simulink model "dspvorbisdec"  (Simulink 8.3)
settings: Solver=FixedStepDiscrete  SolverMode=SingleTasking  StartTime=0.0  StopTime=inf  RelTol=1e-3
PostLoadFcn:
  | hws  = get_param(bdroot,'modelworkspace');
  | dspvorbisdec_SampRt = hws.evalin('dspvorbisdec_OutputSampRt');
  | clear hws;
StopFcn:
  | dspvorbisdec_hws = get_param(bdroot,'modelworkspace');
  | dspvorbisdec_tmp = dspvorbisdec_hws.data;
  | for i = 1:length(dspvorbisdec_tmp)
  |   if strcmp(dspvorbisdec_tmp(i).Name,'dspvorbisdec_OutputSampRt')
  |      if (dspvorbisdec_tmp(i).Value~=dspvorbisdec_SampRt)
  |         dspvorbisdec_hws.assignin('dspvorbisdec_OutputSampRt', dspvorbisdec_SampRt);
  |      end
  |   end
  | end
  | 
  | clear hws dspvorbisdec_tmp i dspvorbisdec_hws;
undefined symbols (not defined in the file or in its folder): blockSize, errordlg, uiwait, warndlg
libraries: simulink x5, dspmtrx3 x3, dspindex x2, dspsigops x1, dspxfrm3 x1, dspmisc x1, dspsnks4 x1, dspsrcs4 x1
(part 3 of 3)

== matlab function Decode All Pages of Data/decodePage/Read Setup Info/Read Setup ==
  data: data input double; codeBooks output double; floor1Data output double; floor1DataLocs output double; resiData output double; numBytes input double; ifUnpack input double; resiDataLocs output double; mapData output double; modeData output double; numChannels input double
function [codeBooks, floor1Data, floor1DataLocs, resiData, resiDataLocs, mapData, modeData] = readSetup(data, numBytes, ifUnpack, numChannels)

codeBooks = uint32(zeros(2*64, 256*30)); % reserve space for codebooks. Standard has capacity for up to 2^32 of them. 
                                         % In this model we assume that number of codebooks cannot be more than 64. Change this quanitity if out of bounds error is experienced
dimLocs = uint32(zeros(256,1));           % Auxiliary array. To specify location of different data in a storage vector
floor1Data = uint32(zeros(256,1));
floor1DataLocs = uint32(zeros(5,32));   % Auxiliary array for floor data vector
resiData = uint32(zeros(256*2,1)); 
resiDataLocs = uint32(zeros(2,8));    % Auxiliary array for residue data vector
mapData = uint32(zeros(5,8));           % Assume we have no more than 2-channel audio
modeData = uint32(zeros(32,1));           % (Same)

persistent tmpPoint;
if isempty(tmpPoint)
	tmpPoint = uint16(0);
end
persistent tmpStorage;
if isempty(tmpStorage)
    tmpStorage = uint32(zeros(15000,1));
end


% Here we check whether compressed setup info header has been buffered completely (ifUnpack==1), 
% or otherwise (ifUnpack==0). 
if (~ifUnpack)
    % If the buffering is not complete yet, then write the first page into temporary buffer
    for w = 1:numBytes
        tmpStorage(tmpPoint+w) = data(w);
    end
    tmpPoint = tmpPoint+numBytes;
else
    % Concatenate the previous page of compressed setup header with the current one and proceed to decoding
    bitstr = logical(false(120000,1));
    for m = 1:tmpPoint
        for t = eml.unroll(1:8)
            bitstr(8*(m-1)+t) = bitget(tmpStorage(m), t);
        end
    end
    for m = 1:numBytes
        for t = eml.unroll(1:8)
            bitstr(8*(m-1)+t+tmpPoint*8) = bitget(data(m), t);
        end
    end
    tmpPoint = uint16(0);    

    %%%%%%%%%%%%%%%%%%%%%%%%%%%%%%%%%%%%%%%%%%%%%%%%%
    %% The code below follows Vorbis decoder spec. %%
    %%%%%%%%%%%%%%%%%%%%%%%%%%%%%%%%%%%%%%%%%%%%%%%%%

    sHead = zeros(3,8);
    tmp = uint8([66 67 86]'); %%%%% Codebook starts with a sync pattern
    for i = uint32(1):uint32(3)
        sHead(i,:) = bitget(tmp(i),1:8);
    end
    syncHead = uint32(reshape(sHead', 24,1));

    %%%%%% Skipping 'Packet type' and 'v o r b i s' fields, 7 bytes total
    bitPoint = uint32(8)*uint32(7) + uint32(1);

    countBooks = uint32(1);
    bitPoint = bitPoint+8;

    % Loop until all codebooks are read 
    totalBooks = uint32(255); %%%%% To be updated
    while (countBooks<=totalBooks)
        codeBook = uint32(zeros(256*30, 1));
    %%%%% We are looking for the sync pattern first
        a = bitPoint;
        while (1==1)
            res=uint32(1);
            i1 = uint32(1):uint32(24);
            i2 = i1+a-1;
            if any(int8(bitstr(i2))-int8(syncHead(i1)))
                res = uint32(0);
            end
            if res; break; end;
            a = a+1;
        end
        if (countBooks ==1)
            bitPoint = a-8; %%%% Skip Sync pattern
            totalBooks = uint32(0);
            for ix = bitPoint:bitPoint+7
                totalBooks = bitset(totalBooks, ix-bitPoint+1, bitstr(ix));
            end
            totalBooks = totalBooks+1;
        end
        bitPoint = a+24;    

        %%% Read codebook dimensions
        for ix = bitPoint:bitPoint+15
            codeBook(1) = bitset(codeBook(1), ix-bitPoint+1, bitstr(ix));            
        end
        bitPoint = bitPoint+16;
        %%% Read codebook length
        %%% Note: can be very long 2^16 bytes. We don't consider such cases here. Assume codebook is short, a couple of kbytes.
        for ix = bitPoint:bitPoint+23
            codeBook(2) = bitset(codeBook(2), ix-bitPoint+1, bitstr(ix));                        
        end
        bitPoint = bitPoint+24;
        bytePoint = uint32(3);

        %%% Read 'ORDERED' flag
        bitPoint=bitPoint+1;
        if bitstr(bitPoint-1)
            curLength = uint32(0);
            for ix = bitPoint:bitPoint+4
                curLength = bitset(curLength, ix-bitPoint+1, bitstr(ix));                            
            end
            bitPoint = bitPoint+5;
            curLength = curLength+1;
            curEntry = uint32(0);
            while(curEntry<codeBook(2))
                ret = uint32(0);
                v = codeBook(2) - curEntry;
                while (v)
                    ret = ret+1;
                    v = bitshift(v,-1);
                end
                %%%%%%%%%%%%%%%%%%        
                number = uint32(0);
                for ix = bitPoint:bitPoint+ret-1;
                    number = bitset(number, ix-bitPoint+1, bitstr(ix));                                                
                end
                bitPoint = bitPoint+ret; % Write entries, ordered
                for k = curEntry:(curEntry+number-1)
                    codeBook(bytePoint) = curLength;
                    bytePoint = bytePoint + 1;
                end
                curEntry = curEntry + number;
                curLength = curLength + 1;
            end
        else
            %%% Read 'SPARSE' flag
            bitPoint=bitPoint+1;       
            if bitstr(bitPoint-1) %% Read entries, sparse
                for i = uint32(1):codeBook(2)
                    bitPoint = bitPoint+1;                
                    if bitstr(bitPoint-1)
                        for ix = bitPoint:bitPoint+4
                            codeBook(bytePoint) = bitset(codeBook(bytePoint), ix-bitPoint+1, bitstr(ix));                                                
                        end
                        bitPoint = bitPoint + 5;
                        codeBook(bytePoint) = codeBook(bytePoint)+1;
                        bytePoint = bytePoint+1;
                    else
                        codeBook(bytePoint) = uint32(0);
                        bytePoint = bytePoint+1;
                    end
                end
            else %% Read entries, not sparse
                for i = uint32(1):codeBook(2)
                    for ix = bitPoint:bitPoint+4
                        codeBook(bytePoint) = bitset(codeBook(bytePoint), ix-bitPoint+1, bitstr(ix));                                                
                    end
                    codeBook(bytePoint) = codeBook(bytePoint)+1;                
                    bitPoint = bitPoint+5;
                    bytePoint = bytePoint+1;
                end
            end
        end

    %%%%%%%%%%%% Read VQ Lookup Header    
        for ix = bitPoint:bitPoint+3;
            codeBook(bytePoint) = bitset(codeBook(bytePoint), ix-bitPoint+1, bitstr(ix));                                                            
        end
        bitPoint = bitPoint + 4;
        bytePoint = bytePoint + 1;
        if codeBook(bytePoint-1)==0
            % Codebook is read, proceed to analysis
        else
            %%%%%%%%% Read VQ Data. Please refer to the decoder spec in 3.2.1.2 for further detail.
            for k = uint32(1):uint32(2)
                for ix = bitPoint:bitPoint+31
                    codeBook(bytePoint) = bitset(codeBook(bytePoint), ix-bitPoint+1, bitstr(ix));                                                                    
                end
                bitPoint = bitPoint + 32;
                bytePoint = bytePoint + 1;
            end            
            for ix = bitPoint:bitPoint+4
                codeBook(bytePoint) = bitset(codeBook(bytePoint), ix-bitPoint+1, bitstr(ix));                                                                
            end            
            bitPoint = bitPoint + 5;

            codeBook(bytePoint+1) = bitshift(codeBook(bytePoint),-4);            
            vqSize = uint32(bitand(codeBook(bytePoint),uint32(15)))+1;
            codeBook(bytePoint) = uint32(vqSize);
            bytePoint = bytePoint + 3;            

            if codeBook(bytePoint-6) == 1
            % The following routines were ported from the original C-code
                vals = uint32(floor(double(codeBook(2))^(1.0/double(codeBook(1))))); %%%%%%% SHOULD BE CHANGED FOR FIXPOINT IMPLEMENTATION
                while (1 == 1)
                    acc = uint32(1);
                    acc1 = uint32(1);
                    for k = uint32(1):codeBook(1)
                        acc = acc*vals;
                        acc1 = acc1*(vals+1);
                    end
                    if (acc<=codeBook(2)) && (acc1>codeBook(2))
                        countBytes = vals; codeBook(bytePoint-1) = vals; break;
                    else
                        if (acc>codeBook(2)); vals = vals - 1;
                        else vals = vals + 1; end
                    end
                end
                 %%%%%%%%%%%%%%%%%%%%%%%%%%%%%%%%%%%%%
            else
                countBytes = codeBook(1)*codeBook(2);
                codeBook(bytePoint-1) = countBytes;
            end 
            for i =uint32(1):countBytes
                for ix = bitPoint:bitPoint+vqSize-1
                    codeBook(bytePoint) = bitset(codeBook(bytePoint), ix-bitPoint+1, bitstr(ix));                                                                    
                end
                bitPoint = bitPoint + vqSize;
                bytePoint = bytePoint + 1;                
            end
        end
    %%%%%%%%%%%% Read place holders
        if (countBooks == totalBooks)
            for ix = bitPoint:bitPoint+5
                codeBook(bytePoint) = bitset(codeBook(bytePoint), ix-bitPoint+1, bitstr(ix));                                                                
            end
            bitPoint = bitPoint + 6;
            codeBook(bytePoint) = codeBook(bytePoint) + 1;
            bitPoint = bitPoint+uint32(16)*codeBook(bytePoint);
        end

    %%%%%%%%%%%%%% Build a codebook tree. Looked up in the original Vorbis C-library %%%%%%%%%%%%%%%
        nozeros = uint32(333333*ones(256*3,1)); % Auxiliary arrays
        cb = uint32(zeros(256*3,1));
        cb2 = uint32(zeros(256*3,1));

        codeBooks(2*countBooks-1, :) = codeBook(:)';

        sparsecount = 0;
        tmp1 = uint32(0);
        for ii = uint32(1):codeBooks(2*countBooks-1,2)
            if (codeBooks(2*countBooks-1, 2+ii)==0)
                sparsecount = sparsecount + 1;
            else
                tmp1 = tmp1+1;
                codeBooks(2*countBooks, codeBooks(2*countBooks-1, 2)+tmp1) = ii;
                nozeros(tmp1) = codeBooks(2*countBooks-1, 2+ii);
                cb2(tmp1) = ii;
            end
        end

        marker = uint32(zeros(33,1));                
        count = uint32(0);
        for ii = uint32(1):codeBooks(2*countBooks-1, 2)
            length1 = codeBooks(2*countBooks-1, 2+ii);
            if (length1>0) 
                entry = marker(length1);
                count = count + 1;
                codeBooks(2*countBooks, count) = entry;
                for j1 = int32(length1):-1:int32(1)
                    if bitand(marker(j1),1)
                        if (j1==1)
                            marker(1) = marker(1) +1;
                        else
                            marker(j1) = uint32(bitshift(marker(j1-1), 1));
                        end
                        break;
                    end
                    marker(j1) = marker(j1) + 1;
                end
                for j = uint32(length1+1):uint32(32) %prune the tree
                    if (bitshift(marker(j), -1)==entry)
                        entry = marker(j);
                        marker(j) = uint32(bitshift(marker(j-1), 1));
                    else
                        break;
                    end
                end
            else
                if(sparsecount==0); count = count + 1; end
            end
        end

        % bitreverse the words
        count = uint32(1);
        for ii=uint32(1):codeBooks(2*countBooks-1, 2)
            temp = uint32(0);
            for j1 = int32(0):int32(codeBooks(2*countBooks-1, 2+ii)-1)
                temp = uint32(bitshift(temp, 1));
                temp = bitor(temp, uint32(bitand(uint32(bitshift(codeBooks(2*countBooks, count), -j1)), 1)));
            end
            if (sparsecount)
                if (codeBooks(2*countBooks-1, 2+ii))
                    codeBooks(2*countBooks, count) = temp;
                    cb(count) = temp;
                    count = count + 1;
                end
            else
                codeBooks(2*countBooks, count) = temp;
                cb(count) = temp;
                count = count + 1;
            end
        end

        % Sort the codewords according to their lengths shortest 
        % come first in order to expedite decoding lookup process
        % Also create index to avoid zero-lengths codewords
        [nozeros1, idx] = sort(nozeros);
        maxLen = uint32(0);
        codeBooks(2*countBooks-1, 256*30-32) = uint32(1);
        for ii = uint32(1):tmp1
            codeBooks(2*countBooks-1, 2+ii) = nozeros1(ii);
            codeBooks(2*countBooks, ii) = cb(idx(ii));
            codeBooks(2*countBooks, codeBooks(2*countBooks-1, 2)+ii) = cb2(idx(ii));    
            if (maxLen<nozeros1(ii))
                if (maxLen>0); codeBooks(2*countBooks-1, 256*30-32+maxLen) = ii; end
                maxLen = nozeros1(ii);
            end
        end
        codeBooks(2*countBooks-1, 256*30-32+maxLen) = tmp1+1;
        for ii = uint32(1):uint32(32)
            if codeBooks(2*countBooks-1, 256*30-32+ii)==0
                codeBooks(2*countBooks-1, 256*30-32+ii)=codeBooks(2*countBooks-1, 256*30-32+ii-1);
            end
        end

        countBooks = countBooks+1; % Codebook has been read, go to the next one    
    end


    %%%%%%%%%%%%%%%%%%%%%%%%%%%%%%%%%%%%%%%%%%%%%%%%%%%%%%%%%%%%%%%%%%%%%%%%%%%%%%%%%%%%%%%%%%%%%%%%%%%%%%
    %%%%%%%%%%%%%%%%%%%%%%%%%%%%%%%% FLOOR SETUP %%%%%%%%%%%%%%%%%%%%%%%%%%%%%%%%%%%%%%%%%%%%%%%%%%%%%%%%%
    %%%%%%%%%%%%%%%%%%%%%%%%%%%%%%%%%%%%%%%%%%%%%%%%%%%%%%%%%%%%%%%%%%%%%%%%%%%%%%%%%%%%%%%%%%%%%%%%%%%%%%

    %%% Following the routines described in  7.2.2. of the spec. Type 1 of the floor is considered.
    bytePoint = uint32(1);

    for ix = bitPoint:bitPoint+5
        floor1Data(bytePoint) = bitset(floor1Data(bytePoint), ix-bitPoint+1, bitstr(ix));                                                        
    end
    floor1Data(bytePoint) = floor1Data(bytePoint)+1;
    bitPoint = bitPoint + 6;
    totalFloor1 = floor1Data(bytePoint);
    bytePoint = bytePoint + 1;

    for countFloor1 = 1:totalFloor1 %% Read totalFloor1 number of Floor 1 setups. 
        for ix = bitPoint:bitPoint+15
            floor1Data(bytePoint) = bitset(floor1Data(bytePoint), ix-bitPoint+1, bitstr(ix));                                                        
        end
        bitPoint = bitPoint + 16;
        bytePoint = bytePoint + 1;

        floor1DataLocs(1, countFloor1) = bytePoint;
        %    Read [floor1_partitions]

        for ix = bitPoint:bitPoint+4
            floor1Data(bytePoint) = bitset(floor1Data(bytePoint), ix-bitPoint+1, bitstr(ix));                                                                    
        end
        bitPoint = bitPoint + 5;
        partitions = floor1Data(bytePoint);
        bytePoint = bytePoint + 1;
        floor1DataLocs(2, countFloor1) = bytePoint;
        offset1 = bytePoint;

        maxClass = uint32(0);
        for  i = uint32(1):partitions
            for ix = bitPoint:bitPoint+3
                floor1Data(bytePoint) = bitset(floor1Data(bytePoint), ix-bitPoint+1, bitstr(ix));                                                                        
            end
            bitPoint = bitPoint + 4;    
            if maxClass<floor1Data(bytePoint); maxClass = floor1Data(bytePoint); end
            bytePoint = bytePoint + 1;    
        end

        maxClass = maxClass + 1; 
        for i = uint32(1):maxClass
            for ix = bitPoint:bitPoint+2
                floor1Data(bytePoint) = bitset(floor1Data(bytePoint), ix-bitPoint+1, bitstr(ix));                                                                        
            end
            bitPoint = bitPoint + 3;        
            dimLocs(i) = bytePoint;
            floor1DataLocs(3, i+16*(countFloor1-1)) = bytePoint;
            floor1Data(bytePoint) = floor1Data(bytePoint) + 1;
            bytePoint = bytePoint + 1;    

            for ix = bitPoint:bitPoint+1
                floor1Data(bytePoint) = bitset(floor1Data(bytePoint), ix-bitPoint+1, bitstr(ix));                                                                        
            end
            bitPoint = bitPoint + 2;            
            bytePoint = bytePoint + 1;

            countBytes = 2^floor1Data(bytePoint-1);
            if (floor1Data(bytePoint-1))
                for ix = bitPoint:bitPoint+7
                    floor1Data(bytePoint) = bitset(floor1Data(bytePoint), ix-bitPoint+1, bitstr(ix));                                                                            
                end
                bitPoint = bitPoint + 8;            
                bytePoint = bytePoint + 1;        
            end
            for j = uint32(1):countBytes
                for ix = bitPoint:bitPoint+7
                    floor1Data(bytePoint) = bitset(floor1Data(bytePoint), ix-bitPoint+1, bitstr(ix));                                                                            
                end
                if (floor1Data(bytePoint)==0) 
                    floor1Data(bytePoint) = 255;
                else
                    floor1Data(bytePoint) = floor1Data(bytePoint) - 1;
                end        
                bitPoint = bitPoint + 8;            
                bytePoint = bytePoint + 1;                
            end
        end

        floor1DataLocs(4, countFloor1) = bytePoint;                    

        for ix = bitPoint:bitPoint+1
            floor1Data(bytePoint) = bitset(floor1Data(bytePoint), ix-bitPoint+1, bitstr(ix));                                                                    
        end
        floor1Data(bytePoint) = floor1Data(bytePoint)+1;
        bitPoint = bitPoint + 2;            
        bytePoint = bytePoint + 1;

        for ix = bitPoint:bitPoint+3
            floor1Data(bytePoint) = bitset(floor1Data(bytePoint), ix-bitPoint+1, bitstr(ix));                                                                    
        end
        bitPoint = bitPoint + 4;            
        rangebits = floor1Data(bytePoint);
        bytePoint = bytePoint + 1;

        floor1DataLocs(5, countFloor1) = bytePoint;  % [floor1_X_locs] 
        floor1Data(bytePoint) = 0;
        bytePoint = bytePoint+1;
        floor1Data(bytePoint) = 2^floor1Data(bytePoint-2);
        bytePoint = bytePoint+1;

        floor1_values = uint32(2);

        for i = uint32(0):(partitions-1)
            countBytes = uint32(floor1Data(dimLocs(floor1Data(offset1+i)+1)));
            floor1_values = floor1_values+uint32(floor1Data(dimLocs(floor1Data(offset1+i)+1)));        

            for k = uint32(1):countBytes
                for ix = bitPoint:bitPoint+uint32(rangebits)-1
                    floor1Data(bytePoint) = bitset(floor1Data(bytePoint), ix-bitPoint+1, bitstr(ix));                                                                            
                end
                bitPoint = bitPoint + uint32(rangebits);
                bytePoint = bytePoint + 1;        
            end
        end
        floor1Data(floor1DataLocs(1, countFloor1)-1) = floor1_values;

        dimLocs = uint32(zeros(256,1));
    end

    %%%%%%%%%%%%%%%%%%%%%%%%%%%%%%%%%%%%%%%%%%%%%%%%%%%%%%%%%%%%%%%%%%%%%%%%%%%%%%%%%%%%%%%%%%%%%%%%%%%%%
    %%%%%%%%%% Read residues %%%%%%%%%%%%%%%%%%%%%%%%%%%%%%%%%%%%%%%%%%%%%%%%%%%%%%%%%%%%%%%%%%%%%%%%%%%%
    %%%%%%%%%%%%%%%%%%%%%%%%%%%%%%%%%%%%%%%%%%%%%%%%%%%%%%%%%%%%%%%%%%%%%%%%%%%%%%%%%%%%%%%%%%%%%%%%%%%%%

    %%% Following the routines described in  8.6.1. of the spec.
    bytePoint = uint32(1);
    for ix = bitPoint:bitPoint+5
        resiData(bytePoint) = bitset(resiData(bytePoint), ix-bitPoint+1, bitstr(ix));                                                                
    end
    resiData(bytePoint) = resiData(bytePoint)+1;
    bitPoint = bitPoint + 6;
    bytePoint = bytePoint + 1;

    for countResi = uint32(1):uint32(resiData(1))

        resiDataLocs(1,countResi) = bytePoint+2;
        for i = uint32(1):uint32(11)
            for ix = bitPoint:bitPoint+7
                resiData(bytePoint) = bitset(resiData(bytePoint), ix-bitPoint+1, bitstr(ix));                                                                                
            end
            bitPoint = bitPoint + 8;
            bytePoint = bytePoint + 1;
        end

        for ix = bitPoint:bitPoint+5
            resiData(bytePoint) = bitset(resiData(bytePoint), ix-bitPoint+1, bitstr(ix));                                                                           
        end
        bitPoint = bitPoint + 6;
        resiData(bytePoint) = resiData(bytePoint)+1;
        residue_classifications = resiData(bytePoint);    
        bytePoint = bytePoint + 1;

        %       [residue_classbook]
        for ix = bitPoint:bitPoint+7
            resiData(bytePoint) = bitset(resiData(bytePoint), ix-bitPoint+1, bitstr(ix));                                                                            
        end
        bitPoint = bitPoint + 8;
        bytePoint = bytePoint + 1;

        acc=uint32(0);
        offset = bytePoint;

        for i =uint32(0):uint32(residue_classifications-1)
            high_bits = uint32(0);
            low_bits = uint32(0);

            % Iterate, read [low_bits]
            for ix = bitPoint:bitPoint+2
                low_bits = bitset(low_bits, ix-bitPoint+1, bitstr(ix));                                                                                
            end
            bitPoint = bitPoint + 3;

            bitPoint = bitPoint + 1;
            if bitstr(bitPoint-1)
                for ix = bitPoint:bitPoint+4
                    high_bits = bitset(high_bits, ix-bitPoint+1, bitstr(ix));                                                                                    
                end
                bitPoint = bitPoint + 5;
            end

            resiData(bytePoint) = uint32(8*high_bits + low_bits); 
            vv = resiData(bytePoint);
            %%%%%%%%%%%%%% icount %%%%%%%%%%%%
            ret = uint32(0);
            while (vv)
                ret = ret + uint32(bitand(vv, 1));
                vv = uint32(bitshift(vv, -1));
            end
            %%%%%%%%%%%%%% end icount %%%%%%%%
            acc = acc + ret;
            bytePoint = bytePoint + 1;
        end
        resiDataLocs(2,countResi) = bytePoint;
        countBytes = acc;

        stages = uint32(0);
        for i = uint32(1):uint32(residue_classifications)
            for j = uint32(1):uint32(8)
                if (bitget(resiData(offset+uint32(i)-1), j)==0)
                    resiData(bytePoint) = 255; % Mark as unused
                    bytePoint = bytePoint + 1;
                else
                    for ix = bitPoint:bitPoint+7
                        resiData(bytePoint) = bitset(resiData(bytePoint), ix-bitPoint+1, bitstr(ix));                                                                                                    
                    end
                    countBytes = countBytes-1;
                    bitPoint = bitPoint + 8;
                    bytePoint = bytePoint + 1;
                    if stages<j; stages = j; end
                    if (countBytes == 0)
                        break;
                    end;
                end
            end
        end

        resiData(resiDataLocs(1,countResi)-1) = stages;
    end

    %%%%%%%%%%%%%%%%%%%%%%%%%%%%%%%%%%%%%%%%%%%%%%%%%%%%%%%%%%%%%%%%%%%%%%%%%%%%%%%%%%%%%%%%%%%%%%%%%%%%
    %%%%%%%%%%%%%%% READ MAPPINGS %%%%%%%%%%%%%%%%%%%%%%%%%%%%%%%%%%%%%%%%%%%%%%%%%%%%%%%%%%%%%%%%%%%%%%
    %%%%%%%%%%%%%%%%%%%%%%%%%%%%%%%%%%%%%%%%%%%%%%%%%%%%%%%%%%%%%%%%%%%%%%%%%%%%%%%%%%%%%%%%%%%%%%%%%%%%

    %%% Following the routines described in  4.2.4.5. of the spec.
    bytePoint = uint32(1);
    for ix = bitPoint:bitPoint+5
        mapData(1,bytePoint) = bitset(mapData(1,bytePoint), ix-bitPoint+1, bitstr(ix));                                                                                    
    end
    mapData(1,bytePoint) = mapData(1,bytePoint)+1;
    bitPoint = bitPoint + 6;


    for count_m = 1:mapData(1,1)
    %   mapping type, needs to be zero
        bitPoint = bitPoint + 17;
        if bitstr(bitPoint-1)
            % vorbis_mapping_submaps
            for ix = bitPoint:bitPoint+3
                mapData(count_m*2,1) = bitset(mapData(count_m*2,1), ix-bitPoint+1, bitstr(ix));                                                                                                    
            end
            mapData(count_m*2,1) = mapData(count_m*2,1)+1;
            bitPoint = bitPoint + 4;
        else
            mapData(1+(count_m-1)*2+1,1) = 1;
        end

        bitPoint = bitPoint + 1;
        if bitstr(bitPoint-1)
            for ix = bitPoint:bitPoint+7
                % vorbis_mapping_coupling_steps
                mapData(count_m*2,2) = bitset(mapData(count_m*2,2), ix-bitPoint+1, bitstr(ix));                                                                                                    
            end        
            mapData(1+(count_m-1)*2+1,2) = mapData(1+(count_m-1)*2+1,2)+1;
            bitPoint = bitPoint+8;
            for q = uint32(1):mapData(1+(count_m-1)*2+1,2) % for each of vorbis_mapping_coupling_steps
                % ilog() function from the original C-library
                ret = uint32(0);
                v = uint32(numChannels)-1;
                while (v)
                    ret = ret+1;
                    v = uint32(bitshift(v,-1));
                end
                %
                count = ret;        
                for ix = bitPoint:bitPoint+count-1
                    % vorbis_mapping_magnitude
                    mapData(count_m*2,3+(q-1)*2) = bitset(mapData(count_m*2,3+(q-1)*2), ix-bitPoint+1, bitstr(ix));                                                                                                                        
                end        
                bitPoint = bitPoint+count;
                for ix = bitPoint:bitPoint+count-1
                    % vorbis_mapping_angle
                    mapData(count_m*2,3+(q-1)*2+1) = bitset(mapData(count_m*2,3+(q-1)*2+1), ix-bitPoint+1, bitstr(ix)); 
                end
                bitPoint = bitPoint+count;
            end
        end
        bitPoint = bitPoint + 2; % read 2 bits, reserved field, currently unused. 

        if (mapData(1+(count_m-1)*2+1,1)>1)
            % read channel multiplex settings
            for q = uint32(1):numChannels
                for ix = bitPoint:bitPoint+3
                    % vorbis_mapping_mux, vector, read numChannel elements
                    mapData(count_m*2+1,q) = bitset(mapData(count_m*2+1,q), ix-bitPoint+1, bitstr(ix)); 
                end
                bitPoint = bitPoint+4;
            end
        end
        for q=uint32(1):mapData(1+(count_m-1)*2+1,1) % for each of vorbis_mapping_submaps
            bitPoint = bitPoint + 8; % read place holder
            for p=uint32(1):uint32(2)
                for ix = bitPoint:bitPoint+7
                    mapData(1+(count_m-1)*2+2,numChannels+(q-1)*2+p) = bitset(mapData(1+(count_m-1)*2+2,numChannels+(q-1)*2+p), ix-bitPoint+1, bitstr(ix));                     
                end
                bitPoint = bitPoint + 8;
            end
        end
    end

    %%%%%%%%%%%%%%%%%%%%%%%%%%%%%%%%%%%%%%%%%%%%%%%%%%%%%%%%%%%%%%%%%%%%%%%%%%%%%%%%%%%%%%%%%%%%%%%%%%%%
    %%%%%%%%%%%%%%% READ MODE SETUP %%%%%%%%%%%%%%%%%%%%%%%%%%%%%%%%%%%%%%%%%%%%%%%%%%%%%%%%%%%%%%%%%%%%
    %%%%%%%%%%%%%%%%%%%%%%%%%%%%%%%%%%%%%%%%%%%%%%%%%%%%%%%%%%%%%%%%%%%%%%%%%%%%%%%%%%%%%%%%%%%%%%%%%%%%

    %%% Following the routines described in 4.2.4.6. of the spec.
    bytePoint = uint32(1);
    for ix = bitPoint:bitPoint+5
        modeData(bytePoint) = bitset(modeData(bytePoint), ix-bitPoint+1, bitstr(ix));                             
    end
    modeData(bytePoint) = modeData(bytePoint)+1;
    bitPoint = bitPoint + 6;
    bytePoint = bytePoint + 1;        

    for count_m = 1:modeData(1)
        modeData(bytePoint) = bitstr(bitPoint);
        bitPoint = bitPoint + 1;
        bytePoint = bytePoint + 1;

        for i = uint32(1):uint32(5)
            for ix = bitPoint:bitPoint+7
                modeData(bytePoint) = bitset(modeData(bytePoint), ix-bitPoint+1, bitstr(ix));                             
            end
            bitPoint = bitPoint + 8;
            bytePoint = bytePoint + 1;                
        end

    end
end

== matlab function Decode All Pages of Data/decodePage/Decode Audio/Decode an Audio Block/Read Packet Header (Spec 4.3.1) ==
  data: overlapPoint output double; leftWindowStart output double; windType output double; data input double; windSize output double; modeData input double; lenLong input double; lenShort input double; stBit output double; mapNumber output double
function [overlapPoint, leftWindowStart, windType, windSize, stBit, mapNumber] ...
    = readPacketHead(data, modeData, lenLong, lenShort)



%%%%%%%% Reading the header of a packet %%%%%%%%%%%%%%%%%%

% ilog() function from the original C-library
bitPoint = uint32(2);

ret = 0;
v = modeData(1)-1;
while (v)
    ret = ret+1;
    v = bitshift(v,-1);
end

leftWindowStart = uint32(0);

buf  = uint8(0);
for i = 1:ret
    buf = bitset(buf, i, bitget(data, bitPoint)); 
    bitPoint = bitPoint + 1;
end

if modeData(2+buf*6)
    windSize = bitshift(uint32(1),lenLong);
    rightWindowStart = windSize/2;                                
    windType = uint8(2);
    prevWindFlag = bitget(data, bitPoint);
    bitPoint = bitPoint + 1;
    if (prevWindFlag==0) 
        windType = windType + 1; 
        leftWindowStart = (windSize-bitshift(uint32(1),lenShort))/4;
    end
    nextWindFlag = bitget(data, bitPoint);
    bitPoint = bitPoint + 1;    
    if (nextWindFlag==0) 
        windType = windType + 2; 
        rightWindowStart = (windSize*3-bitshift(uint32(1),lenShort))/4;
    end    
else
    windSize = bitshift(uint32(1),lenShort);
    rightWindowStart = windSize/2;                                    
    windType = uint8(1);
end

overlapPoint = rightWindowStart-leftWindowStart;
stBit = bitPoint;
mapNumber = modeData(7+buf*6);

== matlab function Decode All Pages of Data/decodePage/Read the Header/Precompute Window Shapes ==
  data: lenLong input double; lenShort input double; wndShapes output double
function wndShapes  = precomputeWindows(lenLong, lenShort)

%wndShapes reference
%Rows #
%1  Small
%2  Large
%3  Large - left-chopped
%4  Laege - right-chopped
%5  Large - both-chopped

wndShapes = zeros(8192, 5);

wndSize = 2^double(lenLong);
window_center = wndSize/2;
left_window_start = 0;
left_window_end = 0;
left_n = 0;
right_window_start = 0;
right_window_end = 0;
right_n = 0;

%   Type 1
left_n=double(2^double(lenShort)/2); 
for q = 1:left_n*2
    wndShapes(q,1)=sin(.5*pi*(sin((q+.5)*.5*pi/left_n))^2);
end

%   Type 2
left_n=double(2^double(lenLong)/2); 
for q = 1:left_n*2
    wndShapes(q,2)=sin(.5*pi*(sin((q+.5)*.5*pi/left_n))^2);
end

%   Type 3
left_window_start = wndSize/4-double(2^double(lenShort)/4);
left_window_end = wndSize/4+double(2^double(lenShort)/4); 
left_n=double(2^double(lenShort)/2); 

right_window_start = window_center;
right_window_end = wndSize;
right_n = wndSize/2;

for q = 1:left_window_start
    wndShapes(q,3) = 0;
end
for q = left_window_start+1:left_window_end
    wndShapes(q,3)=sin(.5*pi*(sin((q+.5-left_window_start)*.5*pi/left_n))^2);
end
for q = left_window_end+1:right_window_start
    wndShapes(q,3) = 1;
end
for q = right_window_start+1:right_window_end
    wndShapes(q,3)=sin(.5*pi*(sin((q+.5-right_window_start)*.5*pi/right_n+.5*pi))^2);
end
for q = right_window_end+1:wndSize
    wndShapes(q,3) = 0;
end

%   Type 4
left_window_start = 0;
left_window_end = window_center;
left_n = wndSize/2;

right_window_start = wndSize*3/4-double(2^double(lenShort)/4);
right_window_end = wndSize*3/4+double(2^double(lenShort)/4); 
right_n=double(2^double(lenShort)/2); 

for q = 1:left_window_start
    wndShapes(q,4) = 0;
end
for q = left_window_start+1:left_window_end
    wndShapes(q,4)=sin(.5*pi*(sin((q+.5-left_window_start)*.5*pi/left_n))^2);
end
for q = left_window_end+1:right_window_start
    wndShapes(q,4) = 1;
end
for q = right_window_start+1:right_window_end
    wndShapes(q,4)=sin(.5*pi*(sin((q+.5-right_window_start)*.5*pi/right_n+.5*pi))^2);
end
for q = right_window_end+1:wndSize
    wndShapes(q,4) = 0;
end

%   Type 5
left_window_start = wndSize/4-double(2^double(lenShort)/4);
left_window_end = wndSize/4+double(2^double(lenShort)/4); 
left_n=double(2^double(lenShort)/2); 

right_window_start = wndSize*3/4-double(2^double(lenShort)/4);
right_window_end = wndSize*3/4+double(2^double(lenShort)/4); 
right_n=double(2^double(lenShort)/2); 

for q = 1:left_window_start
    wndShapes(q,5) = 0;
end
for q = left_window_start+1:left_window_end
    wndShapes(q,5)=sin(.5*pi*(sin((q+.5-left_window_start)*.5*pi/left_n))^2);
end
for q = left_window_end+1:right_window_start
    wndShapes(q,5) = 1;
end
for q = right_window_start+1:right_window_end
    wndShapes(q,5)=sin(.5*pi*(sin((q+.5-right_window_start)*.5*pi/right_n+.5*pi))^2);
end
for q = right_window_end+1:wndSize 
    wndShapes(q,5) = 0;
end
